simulink model "downrightpb"  (R2024b)
settings: Solver=FixedStepAuto  StartTime=0.0  StopTime=10.0  FixedStep=dt  RelTol=1e-3
InitFcn:
  | downrighttest
values from neighbouring files (symbols this model uses):
  A = eye(4) + dt*A    [downrighttest.m]    (also in pendubot_lqr.m)
  B = dt * B    [downrighttest.m]    (also in pendubot_lqr.m)
  dt = 0.01    [EKF_stateFNpb.m]    (also in downrighttest.m; pendubot_lqr.m; simpb_init.m)
  eqb = [-pi/2;0;0;0]    [downrighttest.m]    (also in pendubot_lqr.m = [pi/2;0;0;0]; simpb_init.m = [pi/2;0;0;0])
  initvar = 1e-6    (= 1e-06)    [downrighttest.m]    (also in simpb_init.m)
  K = dlqr(A,B,Q,R)    [downrighttest.m]    (also in pendubot_lqr.m)
  mNoise = diag([mvar,mvar])    [downrighttest.m]    (also in simpb_init.m = diag([mvar,100*mvar]))
  mvar = 10    [downrighttest.m]    (also in simpb_init.m = 0.0001)
  pNoise = diag([pvar,pvar,pvar,pvar])    [downrighttest.m]    (also in simpb_init.m)
  pvar = 0    [downrighttest.m]    (also in simpb_init.m)
  x0 = [-pi/4;0;0;0]    [downrighttest.m]    (also in pendubot_lqr.m = [-pi/2;0;0;0])
libraries: sharedTrackingLibrary x1
settings Model: Creator=heeirthan  LastModifiedBy=heeirthan

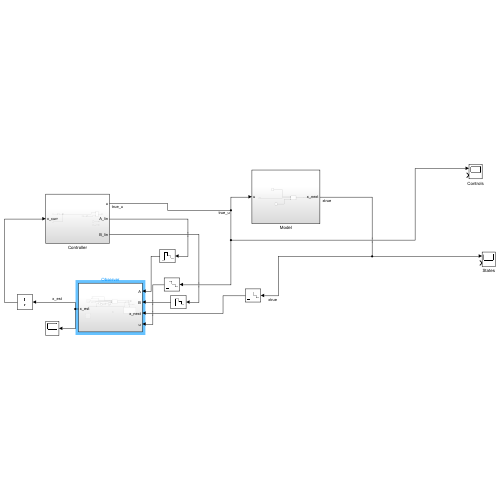
[thumbnail: Simulink's stored preview of the top-level diagram]
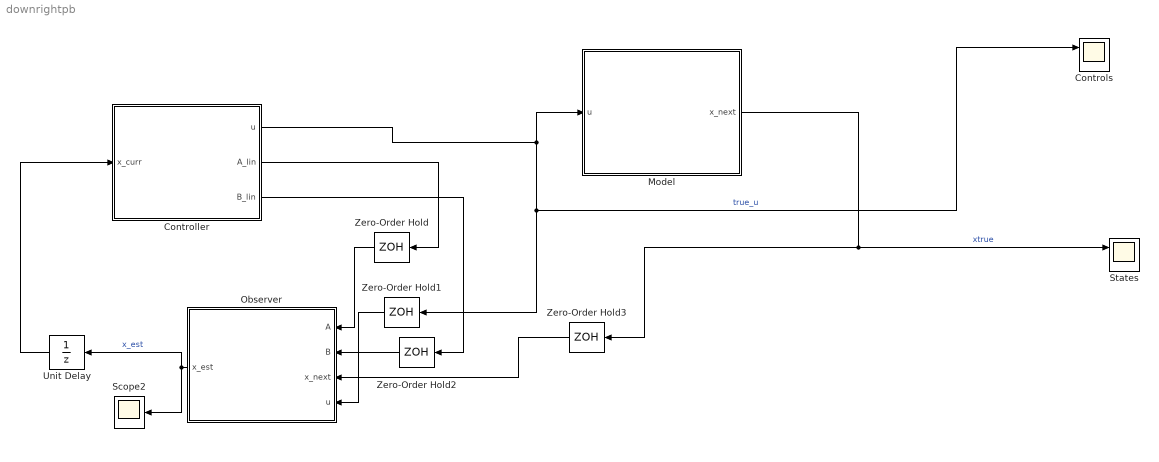
== system downrightpb ==
  Controller : Subsystem
  Controls : Scope  NumInputPorts=2
  Model : Subsystem
  Observer : Subsystem
  Scope2 : Scope
  States : Scope  NumInputPorts=2
  Unit Delay : UnitDelay  InitialCondition=x0  SampleTime=-1  HasFrameUpgradeWarning=on
  Zero-Order Hold{,1..3} (4 alike) : ZeroOrderHold  SampleTime=dt
  wires:
  Controller/1(u) -> Zero-Order Hold1/1, Controls/1, Model/1(u)  "true_u"
  Observer/1(x_est) -> Unit Delay/1, Scope2/1  "x_est"
  Model/1(x_next) -> Zero-Order Hold3/1, States/1  "xtrue"
  Zero-Order Hold1/1 -> Observer/4(u)
  Zero-Order Hold2/1 -> Observer/2(B)
  Zero-Order Hold3/1 -> Observer/3(x_next)
  Zero-Order Hold/1 -> Observer/1(A)
  Controller/2(A_lin) -> Zero-Order Hold/1
  Controller/3(B_lin) -> Zero-Order Hold2/1
  Unit Delay/1 -> Controller/1(x_curr)

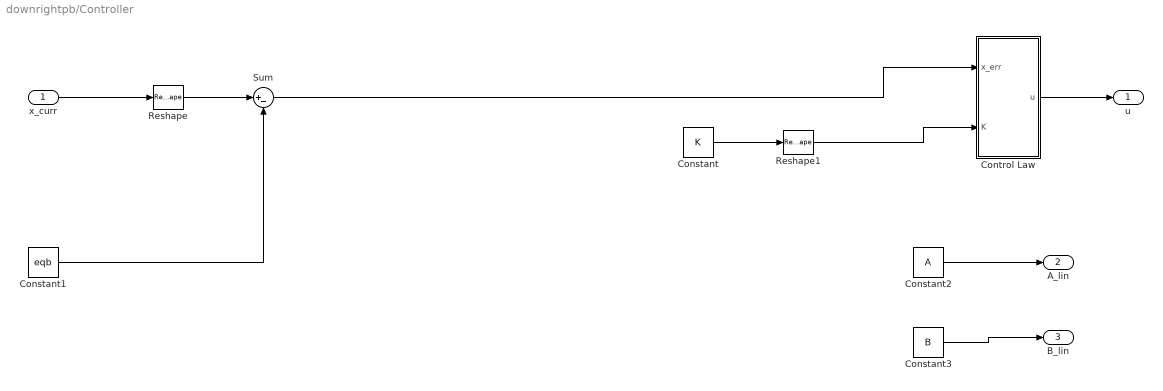
== system downrightpb/Controller ==
  x_curr : Inport
  Constant : Constant  Value=K
  Constant1 : Constant  Value=eqb
  Constant2 : Constant  Value=A
  Constant3 : Constant  Value=B
  Control Law : MATLAB Function  TreatAsAtomicUnit=on
  Reshape : Reshape  OutputDimensionality=Customize  OutputDimensions=[4,1]
  Reshape1 : Reshape  OutputDimensionality=Customize  OutputDimensions=[1,4]
  Sum : Sum  Inputs=|+-
  u : Outport
  A_lin : Outport  Port=2
  B_lin : Outport  Port=3
  wires:
  x_curr/1 -> Reshape/1
  Control Law/1(u) -> u/1
  Constant/1 -> Reshape1/1
  Constant1/1 -> Sum/2
  Sum/1 -> Control Law/1(x_err)
  Constant2/1 -> A_lin/1
  Constant3/1 -> B_lin/1
  Reshape/1 -> Sum/1
  Reshape1/1 -> Control Law/2(K)

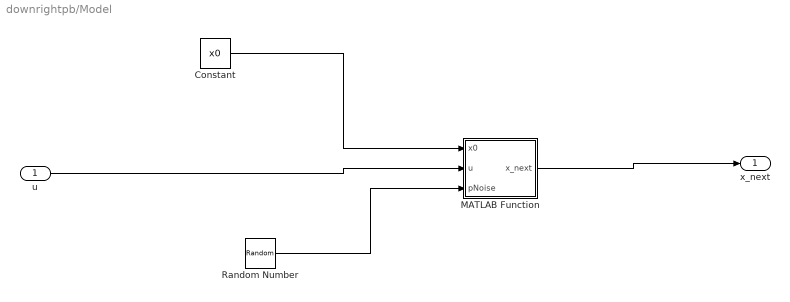
== system downrightpb/Model ==
  u : Inport
  Constant : Constant  Value=x0
  MATLAB Function : MATLAB Function  TreatAsAtomicUnit=on
  Random Number : RandomNumber  Variance=pvar  SampleTime=dt
  x_next : Outport
  wires:
  u/1 -> MATLAB Function/2(u)
  MATLAB Function/1(x_next) -> x_next/1
  Constant/1 -> MATLAB Function/1(x0)
  Random Number/1 -> MATLAB Function/3(pNoise)

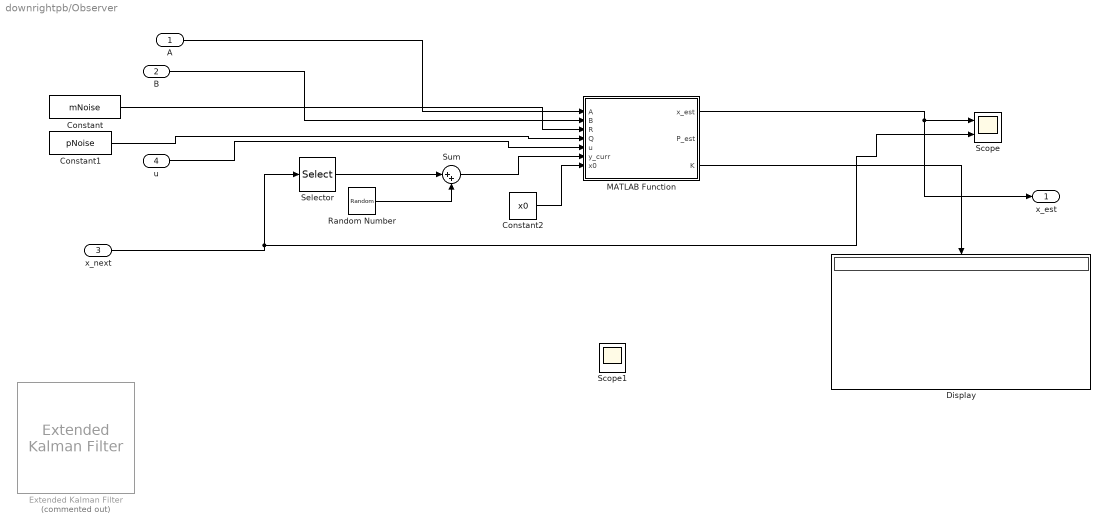
== system downrightpb/Observer ==
  A : Inport
  B : Inport  Port=2
  x_next : Inport  Port=3
  u : Inport  Port=4
  Constant : Constant  Value=mNoise
  Constant1 : Constant  Value=pNoise
  Constant2 : Constant  Value=x0
  Display : Display
  Extended Kalman Filter : sharedTrackingLibrary/Extended Kalman Filter  Commented=on  StateTransitionFcn=EKF_stateFNpb  HasStateTransitionJacobianFcn=off  HasAdditiveProcessNoise=Additive  ProcessNoise=pNoise  HasTimeVaryingProcessNoise=off  HasStateTransitionFcnExtraArgument=1  InitialState=x0  InitialStateCovariance=initvar*eye(4)  MeasurementFcn1=measurementFcn  HasMeasurementJacobianFcn1=off  HasMeasurementEnablePort1=off  HasAdditiveMeasurementNoise1=Additive  MeasurementNoise1=mNoise  HasTimeVaryingMeasurementNoise1=off  HasMeasurementFcnExtraArgument1=0  HasMeasurementWrapping1=off  MeasurementFcn2=myMeasurementFcn  HasMeasurementJacobianFcn2=off  HasMeasurementEnablePort2=off  HasAdditiveMeasurementNoise2=Additive  MeasurementNoise2=1  HasTimeVaryingMeasurementNoise2=off  HasMeasurementFcnExtraArgument2=0  HasMeasurementWrapping2=off  MeasurementFcn3=myMeasurementFcn  HasMeasurementJacobianFcn3=off  HasMeasurementEnablePort3=off  HasAdditiveMeasurementNoise3=Additive  MeasurementNoise3=1  HasTimeVaryingMeasurementNoise3=off  HasMeasurementFcnExtraArgument3=0  HasMeasurementWrapping3=off  MeasurementFcn4=myMeasurementFcn  HasMeasurementJacobianFcn4=off  HasMeasurementEnablePort4=off  HasAdditiveMeasurementNoise4=Additive  MeasurementNoise4=1  HasTimeVaryingMeasurementNoise4=off  HasMeasurementFcnExtraArgument4=0  HasMeasurementWrapping4=off  MeasurementFcn5=myMeasurementFcn  HasMeasurementJacobianFcn5=off  HasMeasurementEnablePort5=off  HasAdditiveMeasurementNoise5=Additive  MeasurementNoise5=1  HasTimeVaryingMeasurementNoise5=off  HasMeasurementFcnExtraArgument5=0  HasMeasurementWrapping5=off  EnableMultirate=off  StateTransitionFcnSampleTime=1  MeasurementFcn1SampleTime=1  MeasurementFcn2SampleTime=1  MeasurementFcn3SampleTime=1  MeasurementFcn4SampleTime=1  MeasurementFcn5SampleTime=1  UseCurrentEstimator=on  OutputStateCovariance=on  DataType=double  SampleTime=dt  NumberOfMeasurements=1
  MATLAB Function : MATLAB Function  TreatAsAtomicUnit=on
  Random Number : RandomNumber  Variance=mvar  SampleTime=dt
  Scope : Scope  NumInputPorts=2
  Scope1 : Scope
  Selector : Selector  InputPortWidth=4  IndexOptions=Index vector (dialog)  Indices=[1 2]  OutputSizes=1
  Sum : Sum  Inputs=|++
  x_est : Outport
  wires:
  x_next/1 -> Selector/1, Scope/2
  u/1 -> MATLAB Function/5(u)
  Selector/1 -> Sum/1
  Sum/1 -> MATLAB Function/6(y_curr)
  Random Number/1 -> Sum/2
  MATLAB Function/1(x_est) -> x_est/1, Scope/1
  Constant1/1 -> MATLAB Function/4(Q)
  MATLAB Function/3(K) -> Display/1
  Constant/1 -> MATLAB Function/3(R)
  A/1 -> MATLAB Function/1(A)
  B/1 -> MATLAB Function/2(B)
  Constant2/1 -> MATLAB Function/7(x0)

== matlab function downrightpb/Model/MATLAB Function ==
  data: x0 input; u input; x_next output; p parameter; pNoise input
function x_next = fcn(x0, u, p, pNoise)
persistent x;
if isempty(x)
    x = x0;
end
dt = 0.01;
x_next = rk4_step(@(xx, uu) dx_pb_lqrreal(0,xx, uu, p), x, u,dt);
x_next(1) = wrapToPi(x_next(1));
x_next(2) = wrapToPi(x_next(2));

x_next = x_next + pNoise;
x = x_next;
end

== matlab function downrightpb/Controller/Control Law ==
  data: x_err input; K input; u output
function u = fcn(x_err,K)
x_err(1) = wrapToPi(x_err(1));
x_err(2) = wrapToPi(x_err(2));

K_max = 50; 
K = max(-K_max, min(K,K_max));
u = 0 - K * x_err;
u_max = 10;
u = max(-u_max, min(u,u_max));

== matlab function downrightpb/Observer/MATLAB Function ==
  data: A input; B input; R input; Q input; u input; y_curr input; x_est output; P_est output; K output; x0 input
function [x_est, P_est, K] = kalman_filter(A,B,R, Q, u, y_curr, x0)

persistent x;
if isempty(x)
    x = x0;
end
persistent P;
if isempty(P)
    P = eye(4)*1e-3;
end

C = [1 0 0 0;
    0 1 0 0];

x_eq = [-pi/2;0;0;0];

x_pred = A*(x-x_eq) + x_eq + B*u;
P_pred = A*P*A' + Q;

K = (P_pred * C') * (C*P_pred*C' + R)^-1;
x_est = x_pred + K*(y_curr - C*x_pred);
%P_est = (eye(4) - K*C)*P_pred;
P_est = ((eye(4)-K*C) * P_pred * (eye(4)-K*C)' + K*R*K');
x = x_est;
P = P_est;
